simulink model "a01_SimTurret"  (R2024a)
settings: Solver=VariableStepAuto  StartTime=0.0  StopTime=10  FixedStep=0.000001  MaxStep=mSim.dTime*0.01  RelTol=mSim.dTime*0.01
PostLoadFcn:
  | a02_SimVariable
undefined symbols (not defined in the file): A02MTRPA, a1st, B01SCHED, b5th, C01ISENS, c7th, CRX1, DC, E03LIM, H01MDE, H01TRT, Init, mDefine, Mech, mSim, MtrPar, Sim, SIM, SimMde
libraries: spsSeriesRLCBranchLib x17, simulink x8, spsCurrentMeasurementLib x7, spsIGBTDiodeLib x7, spsDiodeLib x6, spsControlledVoltageSourceLib x6, spsVoltageMeasurementLib x4, SignalEditorBlockLib x3, spsDCVoltageSourceLib x1, spspowerguiLib x1
(part 1 of 3)
settings Model: VariantConfigurationObject=cfgVariant  SimulationMode=accelerator  NumberOfSteps=10  Creator=MINV  LastModifiedBy=admin
settings SolverCC: MaxConsecutiveZCs=10000  ZeroCrossAlgorithm=Adaptive  AlgebraicLoopSolver=TrustRegion  AutoInsertRateTranBlk=on
settings DataIOCC: InspectSignalLogs=on
settings OptimizationCC: DefaultParameterBehavior=Inlined  UseDivisionForNetSlopeComputation=UseDivisionForReciprocalsOfIntegersOnly  UseFloatMulNetSlope=on  DefaultUnderspecifiedDataType=single  UseSpecifiedMinMax=on  InlineInvariantSignals=on  EnhancedBackFolding=on  PassReuseOutputArgsAs=Individual arguments  ZeroExternalMemoryAtStartup=off  ZeroInternalMemoryAtStartup=off  NoFixptDivByZeroProtection=on  EfficientFloat2IntCast=on  OptimizeBlockOrder=speed  DifferentSizesBufferReuse=on  OptimizationCustomize=off  EfficientTunableParamExpr=on
settings DebuggingCC: SignalInfNanChecking=warning  MaskedZcDiagnostic=none  IgnoredZcDiagnostic=none  IntegerOverflowMsg=none  ParameterPrecisionLossMsg=none  ParameterTunabilityLossMsg=error  UnconnectedInputMsg=warning  UnconnectedOutputMsg=warning  UnconnectedLineMsg=warning  BusObjectLabelMismatch=error  AssertControl=DisableAll  SFUnexpectedBacktrackingDiag=warning  SFNoUnconditionalDefaultTransitionDiag=warning  SFUndirectedBroadcastEventsDiag=error  SFExecutionAtInitializationDiag=none  UnitsInconsistencyMsg=none  ArithmeticOperatorsInVariantConditions=warning
settings HardwareCC: ProdBitPerPointer=32  ProdBitPerSizeT=32  ProdBitPerPtrDiffT=32  ProdLargestAtomicFloat=None  ProdWordSize=32  ProdHWDeviceType=Infineon->TriCore
settings SFSimCC: SimUseLocalCustomCode=off  CompileTimeRecursionLimit=0  EnableRuntimeRecursion=off  MATLABDynamicMemAlloc=off  CustomCodeUndefinedFunction=UseInterfaceOnly
settings RTWCC: Description=Embedded Coder  SystemTargetFile=ert.tlc  GenCodeOnly=on  TemplateMakefile=ert_default_tmf  GenerateReport=on  RTWUseLocalCustomCode=off  CustomHeaderCode="#include \"Define_ASW_Header.h\""  BuildConfiguration=Faster Runs  IncludeHyperlinkInReport=on  LaunchReport=on  GenerateTraceInfo=on  GPUComputeCapability=3.5  DLArmComputeVersion=19.05
settings RTWCC: CustomTerminator=|
  | mVF.VF_cRef_In = 0.0F;
  |     mVF.VF_cRef_In_z = 0.0F;
  |     mVF.VF_Theta = 0.0F;
  |     mVF.V_cRef_In = 0.0F;
  |     mVF.V_cRef_In_z = 0.0F;
  |     mSr.S_Ref_In = 0.0F;
  |     mSEQ.s_Ref_In_z = 0.0F;
  |     mIr.I_cRef_In = 0.0F;
  |     mIr.I_cRef_In_z = 0.0F;
  |     mIr.I_cRef_Limed_z = 0.0F;
  |     rtDW.I_cRef_Limed = 0.0F;
  | 
  |     // V
  |     mSVP.VRef_Max = 0.0F;
  |     mSVP.VRef_Min = 0.0F;
  |     mVr.Vr_Ref_a = 0.0F;
  |     mVr.Vr_Ref_b = 0.0F;
  |     mVr.Vr_Ref_c = 0.0F;
  |     mVn.Vn_Ref_a = 0.0F;
  |     mVn.Vn_Ref_b = 0.0F;
  |     mVn.Vn_Ref_c = 0.0F;
  |     mVe.Ve_Ref_d = 0.0F;
  |     mVe.Ve_Ref_q = 0.0F;
  |     mVe.Ve_d = 0.0F;
  |     mVe.Ve_q = 0.0F;
  |     mVe.Ve_d_z = 0.0F;
  |     mVe.Ve_q_z = 0.0F;
  | 
  |     // IF Initialize
  |     mMC.IF_FREQ = 0.0F;
  |     mMC.IF_Theta = 0.0F;
  | 
  |     // Current Control Initialize
  |     mVe.Ve_d = 0.0F;
  |     mVe.Ve_q = 0.0F;
  |     mVe.Ve_Ref_d = 0.0F;
  |     mVe.Ve_Ref_q = 0.0F;
  |     mTheta.App_sin = 0.0F;
  |     mTheta.App_cos = 0.0F;
  | 
  |     // Sensorless Sequence
  |     if (mWFlag.Pwm_Action == 0U)
  |     {
  |         mSEQ.STEP = 1U;
  |     }
  | 
  |     // Integ
  |     mInteg.Id_Integ = 0.0F;
  |     mInteg.Iq_Integ = 0.0F;
  |     mInteg.I_cRef_Integ = 0.0F;
  |     mEST.We_Integ = 0.0F;
  |     mEST.We_Integ_z = 0.0F;
  |     mEST.Theta_Integ = 0.0F;
  |     mEST.Theta_z = 0.0F;
  |     mVe.Ve_d = 0.0F;
  |     mSr.S_Ref_In = mSEQ.s_Ref_In_z;
settings CodeAppCC: ForceParamTrailComments=on  IgnoreCustomStorageClasses=off  OperatorAnnotations=on  SimulinkDataObjDesc=on  SFDataObjDesc=on  CustomSymbolStrGlobalVar=rt$N$M  CustomSymbolStrType=$N$M  CustomSymbolStrFcn=$N$M$F  CustomSymbolStrMacro=$N$M  DefineNamingRule=UpperCase  ParamNamingRule=UpperCase  InsertBlockDesc=on  EnableCustomComments=on
settings ERTTargetCC: GenerateSampleERTMain=on  InlinedParameterPlacement=NonHierarchical  ERTCustomFileTemplate=example_file_process.tlc
settings ConfigComp: CovScope=ReferencedModels  CovIncludeTopModel=off  CovMetricSettings=dw  CovSaveCumulativeToWorkspaceVar=on  CovSaveSingleToWorkspaceVar=on  CovExternalEMLEnable=off  PSModelRefIgnoreList=[]  PSEnableModelRefIgnoreList=off  PSModelRefMinMaxVerif=CheckAndConstrain  PSAutoStubLUT=on  DVTestSuiteOptimization=CombinedObjectives (Nonlinear Extended)  DVRebuildModelRepresentation=Always
settings SimscapeCC: SimscapeNormalizeSystem=off

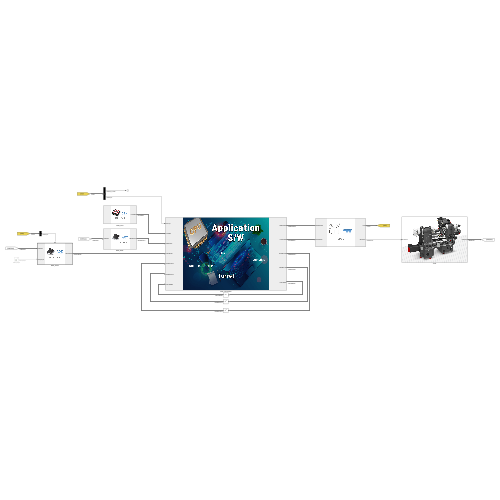
[thumbnail: Simulink's stored preview of the top-level diagram]
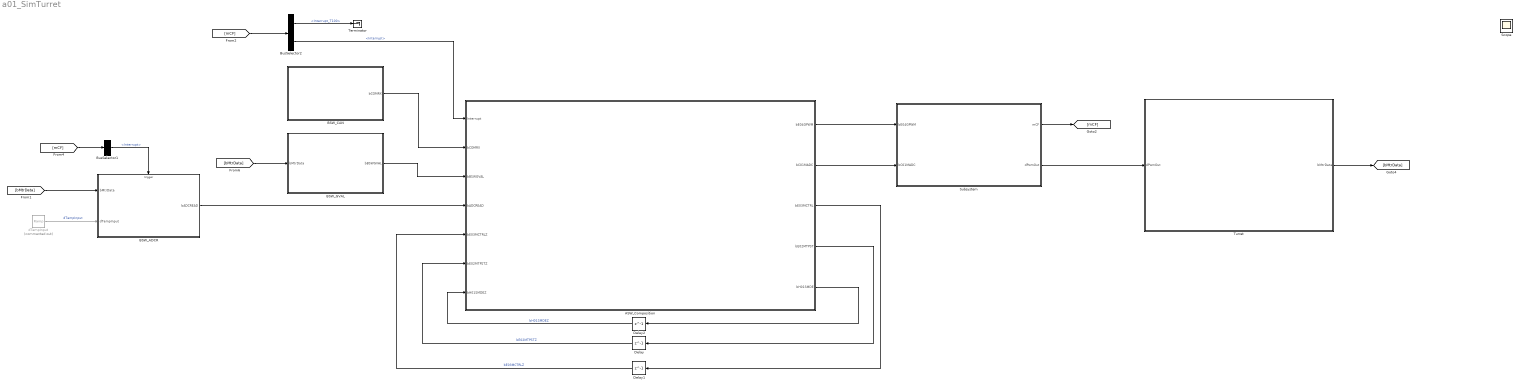
== system a01_SimTurret ==
  ASW_Composition : Subsystem
      mask Display: image('AppSW.png');
  BSW_ADCR : Subsystem
      mask Display: image('ADCREAD_2.png');
  BSW_CAN : Subsystem
      mask Display: image('CANRX1.png');
  BSW_GVAL : Subsystem
      mask Display: image('BSW.png');
  BusSelector1 : BusSelector  OutputSignals=Interrupt
  BusSelector2 : BusSelector  OutputSignals=Interrupt_T100,Interrupt
  Delay : Delay  DelayLength=1
  Delay1 : Delay  DelayLength=1
  Delay2 : Delay  DelayLength=1
  Subsystem : Subsystem
      mask Display: image('ePWM.png');
  Terminator : Terminator
  Turret : Subsystem
      mask Display: image('Turret_2.png');
  dTempInput : simulink/Sources/Ramp  Commented=on  slope=-4096*1.5  start=0  InitialOutput=2048
  Scope : Scope
  wires:
  Turret/1(bMtrData) -> [bMtrData]
  Subsystem/1(mCF) -> [mCF]
  Subsystem/2(dPwmOut) -> Turret/1(dPwmOut)
  [bMtrData] -> BSW_ADCR/1(bMtrData)
  BSW_ADCR/1(bADCREAD) -> ASW_Composition/4(bADCREAD)
  [mCF] -> BusSelector1/1
  BusSelector1/1 -> BSW_ADCR/Trigger  "<Interrupt>"
  dTempInput/1 -> BSW_ADCR/2(dTempInput)  "dTempInput"
  [bMtrData] -> BSW_GVAL/1(bMtrData)
  ASW_Composition/1(bE04GPWM) -> Subsystem/1(bE04GPWM)
  ASW_Composition/2(bC01MADC) -> Subsystem/2(bC01MADC)
  BSW_GVAL/1(bBSWGVAL) -> ASW_Composition/3(bBSWGVAL)
  ASW_Composition/4(bE02MTPST) -> Delay/1
  Delay/1 -> ASW_Composition/6(bE02MTPSTZ)  "bE02MTPSTZ"
  ASW_Composition/3(bE03MCTRL) -> Delay1/1
  Delay1/1 -> ASW_Composition/5(bE03MCTRLZ)  "bE03MCTRLZ"
  BusSelector2/1 -> Terminator/1  "<Interrupt_T100>"
  [mCF] -> BusSelector2/1
  BSW_CAN/1(bCOMRX) -> ASW_Composition/2(bCOMRX)
  ASW_Composition/5(bH01SMDE) -> Delay2/1
  Delay2/1 -> ASW_Composition/7(bH01SMDEZ)  "bH01SMDEZ"
  BusSelector2/2 -> ASW_Composition/1(Interrupt)  "<Interrupt>"

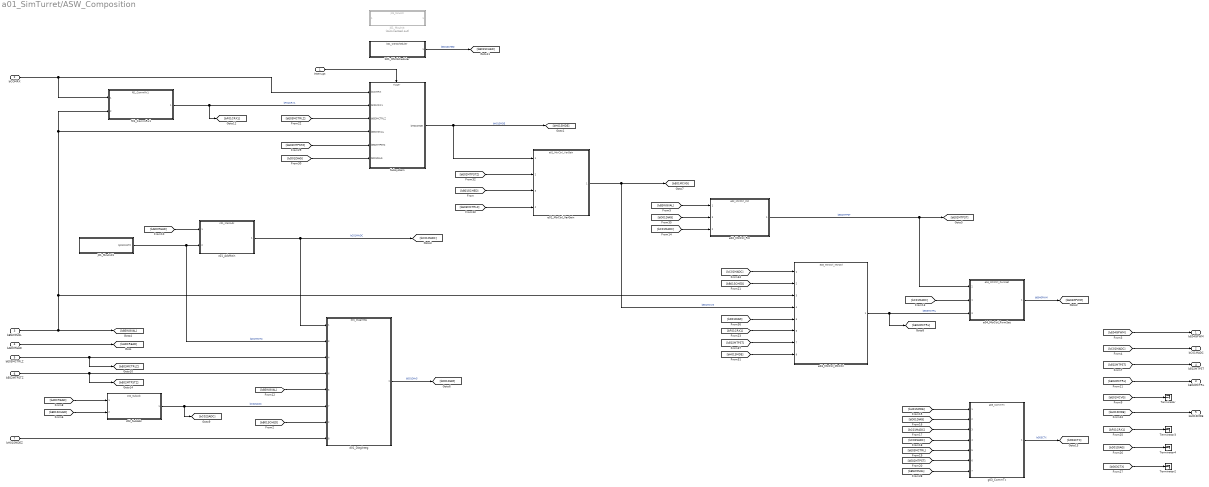
== system a01_SimTurret/ASW_Composition ==
  Interrupt : Inport
  bCOMRX : Inport  Port=2
  bBSWGVAL : Inport  Port=3
  bADCREAD : Inport  Port=4
  bE03MCTRLZ : Inport  Port=5
  bE02MTPSTZ : Inport  Port=6
  bH01SMDEZ : Inport  Port=7
  Subsystem : Subsystem
  Terminator{,2..4} (4 alike) : Terminator
  b01_OSnScheduler : ModelReference  ModelNameDialog=b01_OSnScheduler.slx  SimulationMode=Normal  ModelReferenceVersion=7.234
  c01_AdcMain : ModelReference  ModelNameDialog=c01_MainAdc.slx  SimulationMode=Normal  ModelReferenceVersion=7.199
  c02_SubAdc : ModelReference  ModelNameDialog=c02_SubAdc.slx  SimulationMode=Normal  ModelReferenceVersion=7.333
  d01_Diaglnteg : ModelReference  ModelNameDialog=d01_Diaglnteg.slx  SimulationMode=Normal  ModelReferenceVersion=7.634
      settings: PortSchema="{\"entries\":[{\"content\":{\"sides\":[{\"content\":{\"connectorIds\":[\"In1\",\"In3\",\"In4\",\"In6\",\"In5\",\"In7\",\"In2\",\"In8\"]},\"type\":\"ConnectorPlacement.EquallySpacedRectSide\",\"uuid\":\"173800be-f5dc-4729-8663-94e6b8956988\"},{\"content\":{\"connectorIds\":[\"Out1\"],\"side\":\"RIGHT\"},\"type\":\"ConnectorPlacement.EquallySpacedRectSide\",\"uuid\":\"97fb1ab8-9be5-42b7-b1bf-027aede52d4b\"},{\"content\":{\"side\":\"TOP\"},\"type\":\"ConnectorPlacement.EquallySpacedRectSide\",\"uuid\":\"2e8adbd0-ac2b-453b-9e60-9040db9b7bc5\"}]},\"type\":\"ConnectorPlacement.EquallySpacedConnector\",\"uuid\":\"3d6050df-28eb-4a7c-b004-dbb78ba9bd4d\"}],\"packageUris\":[\"http://schema.mathworks.com/mf0/Connector/R2020b\"],\"version\":\"1.0\"}"
  e01_MtrCtrl_VarGain : ModelReference  ModelNameDialog=e01_MtrCtrl_VarGain.slx  SimulationMode=Normal  ModelReferenceVersion=7.579
  e02_MtrCtrl_Pst : ModelReference  ModelNameDialog=e02_MtrCtrl_Pst.slx  SimulationMode=Normal  ModelReferenceVersion=7.578
      settings: PortSchema="{\"entries\":[{\"content\":{\"sides\":[{\"content\":{\"connectorIds\":[\"In1\",\"In3\",\"In2\"]},\"type\":\"ConnectorPlacement.EquallySpacedRectSide\",\"uuid\":\"f113863a-975d-4050-818f-27abf814cfb5\"},{\"content\":{\"connectorIds\":[\"Out1\"],\"side\":\"RIGHT\"},\"type\":\"ConnectorPlacement.EquallySpacedRectSide\",\"uuid\":\"6686929e-870a-4175-88de-c3673796ef3d\"},{\"content\":{\"side\":\"TOP\"},\"type\":\"ConnectorPlacement.EquallySpacedRectSide\",\"uuid\":\"709e4a9d-e71c-4478-b192-cfc6b94393ff\"}]},\"type\":\"ConnectorPlacement.EquallySpacedConnector\",\"uuid\":\"0b953766-3c3a-41c3-a306-f68929d7ac7c\"}],\"packageUris\":[\"http://schema.mathworks.com/mf0/Connector/R2020b\"],\"version\":\"1.0\"}"
  e03_MtrCtrl_MtrCtrl : ModelReference  ModelNameDialog=e03_MtrCtrl_MtrCtrl.slx  SimulationMode=Normal  ModelReferenceVersion=7.948
  e04_MtrCtrl_PwmSet : ModelReference  ModelNameDialog=e04_MtrCtrl_PwmSet.slx  SimulationMode=Normal  ModelReferenceVersion=7.212
      settings: PortSchema="{\"entries\":[{\"content\":{\"sides\":[{\"content\":{\"connectorIds\":[\"In2\",\"In1\",\"In3\"]},\"type\":\"ConnectorPlacement.EquallySpacedRectSide\",\"uuid\":\"f113863a-975d-4050-818f-27abf814cfb5\"},{\"content\":{\"connectorIds\":[\"Out1\"],\"side\":\"RIGHT\"},\"type\":\"ConnectorPlacement.EquallySpacedRectSide\",\"uuid\":\"6686929e-870a-4175-88de-c3673796ef3d\"},{\"content\":{\"side\":\"TOP\"},\"type\":\"ConnectorPlacement.EquallySpacedRectSide\",\"uuid\":\"709e4a9d-e71c-4478-b192-cfc6b94393ff\"}]},\"type\":\"ConnectorPlacement.EquallySpacedConnector\",\"uuid\":\"0b953766-3c3a-41c3-a306-f68929d7ac7c\"}],\"packageUris\":[\"http://schema.mathworks.com/mf0/Connector/R2020b\"],\"version\":\"1.0\"}"
  f01_CommRx1 : ModelReference  ModelNameDialog=f01_CommRx1.slx  SimulationMode=Normal  ModelReferenceVersion=7.313
  g03_CommTx : ModelReference  ModelNameDialog=g03_CommTx.slx  SimulationMode=Normal  ModelReferenceVersion=7.362
  j01_McuInit : ModelReference  Commented=on  ModelNameDialog=j01_McuInit.slx  SimulationMode=Normal  ModelReferenceVersion=7.616
  j01_McuInit1 : Subsystem
  bE04GPWM : Outport
  bC01MADC : Outport  Port=2
  bE03MCTRL : Outport  Port=3
  bE02MTPST : Outport  Port=4
  bH01SMDE : Outport  Port=5
  wires:
  c01_AdcMain/1 -> [bC01MADC], d01_Diaglnteg/1  "bC01MADC"
  b01_OSnScheduler/1 -> [bB01SCHED]  "bB01SCHED"
  bADCREAD/1 -> [bADCREAD]
  c02_SubAdc/1 -> [bC02SADC], d01_Diaglnteg/7  "bC02SADC"
  e04_MtrCtrl_PwmSet/1 -> [bE04GPWM]  "bE04GPWM"
  [bE04GPWM] -> bE04GPWM/1
  [bC01MADC] -> bC01MADC/1
  e02_MtrCtrl_Pst/1 -> e04_MtrCtrl_PwmSet/2, [bE02MTPST]  "bE02MTPST"
  [bBSWGVAL] -> e02_MtrCtrl_Pst/1
  d01_Diaglnteg/1 -> [bD01DIAG]  "bD01DIAG"
  [bE02MTPST] -> bE02MTPST/1
  e01_MtrCtrl_VarGain/1 -> e03_MtrCtrl_MtrCtrl/4, [bE01MCVG]  "bE01MCVG"
  [bE01MCVG] -> Terminator/1
  bE03MCTRLZ/1 -> [bE03MCTRLZ], d01_Diaglnteg/4
  [bE03MCTRL] -> bE03MCTRL/1
  bE02MTPSTZ/1 -> [bE02MTPSTZ], d01_Diaglnteg/6
  bBSWGVAL/1 -> f01_CommRx1/2, Subsystem/4(bBSWGVAL), e03_MtrCtrl_MtrCtrl/3, [bBSWGVAL]
  [bB01SCHED] -> e01_MtrCtrl_VarGain/3
  [bB01SCHED] -> d01_Diaglnteg/2
  [bB01SCHED] -> c02_SubAdc/2
  [bADCREAD] -> c02_SubAdc/1
  [bADCREAD] -> c01_AdcMain/1
  [bBSWGVAL] -> d01_Diaglnteg/5
  [bC01MADC] -> e04_MtrCtrl_PwmSet/1
  [bC01MADC] -> e02_MtrCtrl_Pst/2
  Subsystem/1(bH01SMDE) -> e01_MtrCtrl_VarGain/1, [bH01SMDE]  "bH01SMDE"
  j01_McuInit1/1(bJ01MINITZ) -> c01_AdcMain/2, d01_Diaglnteg/3  "bJ01MINITZ"
  bCOMRX/1 -> Subsystem/1(bCOMRX), f01_CommRx1/1
  [bF01CRX1] -> e03_MtrCtrl_MtrCtrl/6
  g03_CommTx/1 -> [bG03CTX]  "bG03CTX"
  [bH01SMDE] -> g03_CommTx/1
  [bD01DIAG] -> g03_CommTx/2
  [bC01MADC] -> g03_CommTx/3
  [bE02MTPST] -> g03_CommTx/6
  [bE03MCTRL] -> g03_CommTx/5
  [bC02SADC] -> g03_CommTx/4
  e03_MtrCtrl_MtrCtrl/1 -> e04_MtrCtrl_PwmSet/3, [bE03MCTRL]  "bE03MCTRL"
  [bB01SCHED] -> e03_MtrCtrl_MtrCtrl/2
  [bE03MCTRLZ] -> Subsystem/3(bE03MCTRLZ)
  f01_CommRx1/1 -> [bF01CRX1], Subsystem/2(bF01CRX1)  "bF01CRX1"
  [bH01SMDE] -> bH01SMDE/1
  [bF01CRX1] -> Terminator3/1
  [bD01DIAG] -> Terminator4/1
  [bG03CTX] -> Terminator2/1
  [bBSWGVAL] -> g03_CommTx/7
  [bE02MTPSTZ] -> Subsystem/5(bE02MTPSTZ)
  [bD01DIAG] -> Subsystem/6(bD01DIAG)
  [bH01SMDE] -> e03_MtrCtrl_MtrCtrl/8
  [bE02MTPSTZ] -> e01_MtrCtrl_VarGain/2
  [bE03MCTRLZ] -> e01_MtrCtrl_VarGain/4
  [bC01MADC] -> e03_MtrCtrl_MtrCtrl/1
  [bD01DIAG] -> e02_MtrCtrl_Pst/3
  [bD01DIAG] -> e03_MtrCtrl_MtrCtrl/5
  [bE02MTPST] -> e03_MtrCtrl_MtrCtrl/7
  bH01SMDEZ/1 -> d01_Diaglnteg/8
  Interrupt/1 -> Subsystem/Trigger

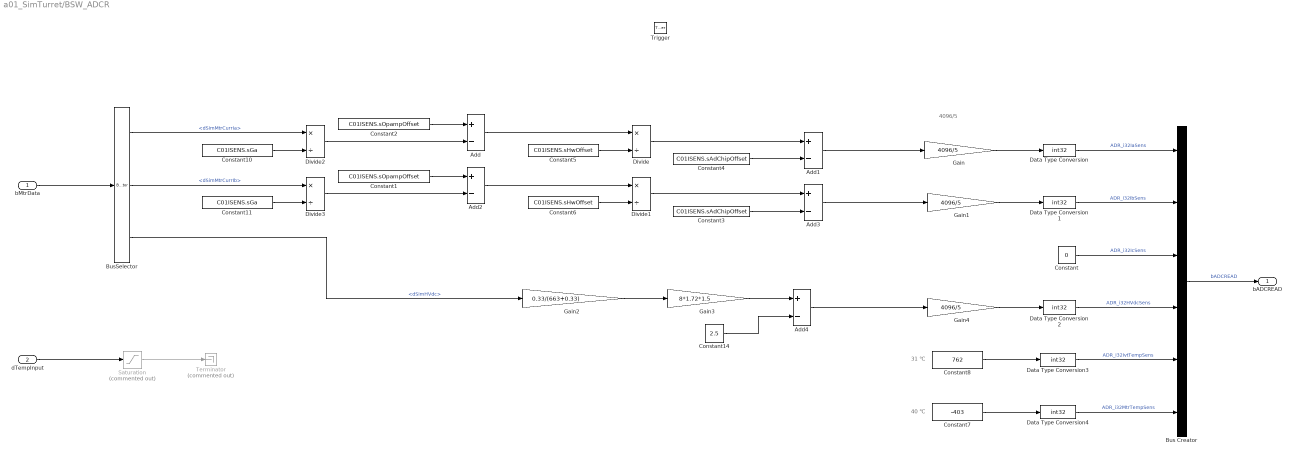
== system a01_SimTurret/BSW_ADCR ==
  note: 4096/5
  note: 40 ℃
  note: 31 ℃
  bMtrData : Inport
  dTempInput : Inport  Port=2
  Trigger : TriggerPort  VariantControl=(inherit)  PortDimensions=1
  Add{,1..4} (5 alike) : Sum  Inputs=+-
  Bus Creator : BusCreator  Inputs=6  OutDataTypeStr=Bus: X_ADCREAD
  BusSelector : BusSelector  OutputSignals=dSimPwrStack.dSimMtrCurrIa,dSimPwrStack.dSimMtrCurrIb,dSimPwrStack.dSimHVdc
  Constant : Constant  Value=0  OutDataTypeStr=int32
  Constant1 : Constant  Value=C01ISENS.sOpampOffset
  Constant10 : Constant  Value=C01ISENS.sGa  OutDataTypeStr=single
  Constant11 : Constant  Value=C01ISENS.sGa  OutDataTypeStr=single
  Constant14 : Constant  Value=2.5
  Constant2 : Constant  Value=C01ISENS.sOpampOffset
  Constant3 : Constant  Value=C01ISENS.sAdChipOffset  OutDataTypeStr=single
  Constant4 : Constant  Value=C01ISENS.sAdChipOffset  OutDataTypeStr=single
  Constant5 : Constant  Value=C01ISENS.sHwOffset  OutDataTypeStr=single
  Constant6 : Constant  Value=C01ISENS.sHwOffset  OutDataTypeStr=single
  Constant7 : Constant  Value=-403
  Constant8 : Constant  Value=762
  Data Type Conversion{,1..4} (5 alike) : DataTypeConversion  OutDataTypeStr=int32  SaturateOnIntegerOverflow=off  RndMeth=Floor
  Divide{,1..3} (4 alike) : Product  Inputs=*/
  Gain : Gain  Gain=4096/5
  Gain1 : Gain  Gain=4096/5
  Gain2 : Gain  Gain=0.33/(663+0.33)
  Gain3 : Gain  Gain=8*1.72*1.5
  Gain4 : Gain  Gain=4096/5
  Saturation : Saturate  Commented=on  UpperLimit=24  LowerLimit=23
  Terminator : Terminator  Commented=on
  bADCREAD : Outport
  wires:
  Constant5/1 -> Divide/2
  Constant2/1 -> Add/1
  Divide/1 -> Add1/1
  Constant4/1 -> Add1/2
  Gain/1 -> Data Type Conversion/1
  Add/1 -> Divide/1
  bMtrData/1 -> BusSelector/1
  BusSelector/1 -> Divide2/1  "<dSimMtrCurrIa>"
  BusSelector/2 -> Divide3/1  "<dSimMtrCurrIb>"
  Bus Creator/1 -> bADCREAD/1  "bADCREAD"
  Data Type Conversion/1 -> Bus Creator/1  "ADR_i32IaSens"
  Constant1/1 -> Add2/1
  Gain1/1 -> Data Type Conversion1/1
  Add2/1 -> Divide1/1
  Constant3/1 -> Add3/2
  Constant6/1 -> Divide1/2
  Divide1/1 -> Add3/1
  Data Type Conversion1/1 -> Bus Creator/2  "ADR_i32IbSens"
  Constant/1 -> Bus Creator/3  "ADR_i32IcSens"
  Gain4/1 -> Data Type Conversion2/1
  Data Type Conversion3/1 -> Bus Creator/5  "ADR_i32IvtTempSens"
  Data Type Conversion4/1 -> Bus Creator/6  "ADR_i32MtrTempSens"
  Constant10/1 -> Divide2/2
  Divide2/1 -> Add/2
  Constant11/1 -> Divide3/2
  Divide3/1 -> Add2/2
  BusSelector/3 -> Gain2/1  "<dSimHVdc>"
  Gain2/1 -> Gain3/1
  Gain3/1 -> Add4/1
  Constant14/1 -> Add4/2
  Add4/1 -> Gain4/1
  Data Type Conversion2/1 -> Bus Creator/4  "ADR_i32HVdcSens"
  dTempInput/1 -> Saturation/1
  Saturation/1 -> Terminator/1
  Constant7/1 -> Data Type Conversion4/1
  Constant8/1 -> Data Type Conversion3/1
  Add1/1 -> Gain/1
  Add3/1 -> Gain1/1

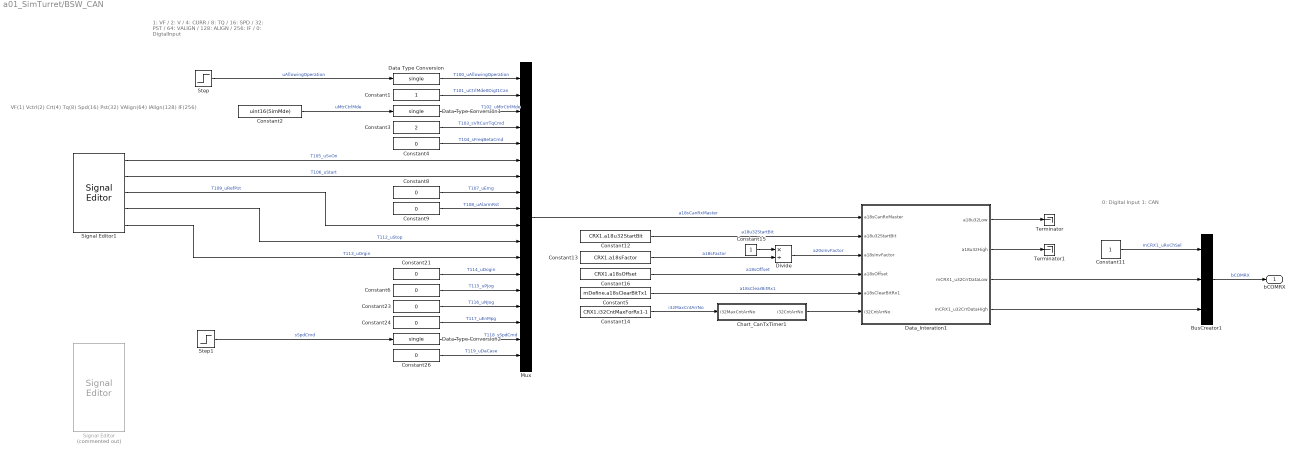
== system a01_SimTurret/BSW_CAN ==
  note: VF(1) Vctrl(2) Crt(4) Tq(8) Spd(16) Pst(32) VAlign(64) IAlign(128) IF(256)
  note: 1: VF / 2: V / 4: CURR / 8: TQ / 16: SPD /
      | 32: PST / 64: VALIGN / 128: ALIGN /
      | 256: IF / 0: DigtalInput
  note: 0: Digital Input
      | 1: CAN
  BusCreator1 : BusCreator  Inputs=3  OutDataTypeStr=Bus: X_COMRX
  Chart_CanTxTimer1 : Stateflow chart  TreatAsAtomicUnit=on
  Constant1 : Constant  OutDataTypeStr=single
  Constant11 : Constant  OutDataTypeStr=uint16
  Constant12 : Constant  Value=CRX1.a18u32StartBit
  Constant13 : Constant  Value=CRX1.a18sFactor
  Constant14 : Constant  Value=CRX1.i32CntMaxForRx1-1  OutDataTypeStr=int32
  Constant15 : Constant  OutDataTypeStr=single
  Constant16 : Constant  Value=CRX1.a18sOffset
  Constant2 : Constant  Value=uint16(SimMde)  OutDataTypeStr=single
  Constant{4,6,8..9,21,23..24,26} (8 alike) : Constant  Value=0  OutDataTypeStr=single
  Constant3 : Constant  Value=2  OutDataTypeStr=single
  Constant5 : Constant  Value=mDefine.a18sClearBitTx1
  Data Type Conversion : DataTypeConversion  OutDataTypeStr=single  SaturateOnIntegerOverflow=off  RndMeth=Floor
  Data Type Conversion1 : DataTypeConversion  OutDataTypeStr=single  SaturateOnIntegerOverflow=off  RndMeth=Floor
  Data Type Conversion2 : DataTypeConversion  OutDataTypeStr=single  SaturateOnIntegerOverflow=off  RndMeth=Floor
  Data_Interation1 : Stateflow chart  TreatAsAtomicUnit=on
      settings: RTWSystemCode=Inline
  Divide : Product  Inputs=*/  OutDataTypeStr=single
  Mux : Mux  Inputs=18
  Signal Editor : SignalEditorBlockLib/Signal Editor  Commented=on  FileName=TestOrigin3.mat  ActiveScenario=Scenario  ActiveSignal=Origin  IsBus=off  OutputBusObjectStr=Bus: BusObject  SampleTime=0  Interpolate=off  ZeroCross=off  OutputAfterFinalValue=Setting to zero  Unit=inherit  PreserveSignalName=on  ApplySigPropsToAllScenarios=on  ApplySigPropsToAllSignals=off
  Signal Editor1 : SignalEditorBlockLib/Signal Editor  FileName=TestOrigin4.mat  ActiveScenario=Scenario  ActiveSignal=Origin  IsBus=off  OutputBusObjectStr=Bus: BusObject  SampleTime=0  Interpolate=off  ZeroCross=off  OutputAfterFinalValue=Setting to zero  Unit=inherit  PreserveSignalName=on  ApplySigPropsToAllScenarios=on  ApplySigPropsToAllSignals=off
  Step : Step  After=0  SampleTime=0
  Step1 : Step  Time=3  Before=-500  After=1000  SampleTime=0
  Terminator : Terminator
  Terminator1 : Terminator
  bCOMRX : Outport
  wires:
  Constant5/1 -> Data_Interation1/5(a18sClearBitRx1)  "a18sClearBitRx1"
  Data_Interation1/4(mCRX1_u32CrrDataHigh) -> BusCreator1/3
  Constant13/1 -> Divide/2  "a18sFactor"
  Mux/1 -> Data_Interation1/1(a18sCanRxMaster)  "a18sCanRxMaster"
  Constant14/1 -> Chart_CanTxTimer1/1(i32MaxCntArrNo)  "i32MaxCntArrNo"
  Divide/1 -> Data_Interation1/3(a18sInvFactor)  "a20sInvFactor"
  Data_Interation1/1(a18u32Low) -> Terminator/1
  Data_Interation1/2(a18u32High) -> Terminator1/1
  Constant12/1 -> Data_Interation1/2(a18u32StartBit)  "a18u32StartBit"
  Data_Interation1/3(mCRX1_u32CrrDataLow) -> BusCreator1/2
  Constant16/1 -> Data_Interation1/4(a18sOffset)  "a18sOffset"
  Chart_CanTxTimer1/1(i32CntArrNo) -> Data_Interation1/6(i32CntArrNo)
  BusCreator1/1 -> bCOMRX/1  "bCOMRX"
  Constant15/1 -> Divide/1
  Constant11/1 -> BusCreator1/1  "mCRX1_uRxChSel"
  Data Type Conversion/1 -> Mux/1  "T100_uAllowingOperation"
  Constant1/1 -> Mux/2  "T101_uCtrlMde0Digt1Can"
  Constant2/1 -> Data Type Conversion1/1  "uMtrCtrlMde"
  Constant3/1 -> Mux/4  "T103_sVltCurrTqCmd"
  Constant8/1 -> Mux/8  "T107_uEmg"
  Signal Editor1/2 -> Mux/7  "T106_uStart"
  Signal Editor1/1 -> Mux/6  "T105_uSvOn"
  Constant4/1 -> Mux/5  "T104_sFreqBetaCmd"
  Signal Editor1/4 -> Mux/11  "T112_uStop"
  Signal Editor1/5 -> Mux/12  "T113_uOrgin"
  Constant21/1 -> Mux/13  "T114_uDogin"
  Constant6/1 -> Mux/14  "T115_uPJog"
  Signal Editor1/3 -> Mux/10  "T109_uRefPst"
  Constant9/1 -> Mux/9  "T108_uAlarmRst"
  Constant23/1 -> Mux/15  "T116_uNJog"
  Constant26/1 -> Mux/18  "T119_uDaCase"
  Constant24/1 -> Mux/16  "T117_uEnMpg"
  Data Type Conversion1/1 -> Mux/3  "T102_uMtrCtrlMde"
  Data Type Conversion2/1 -> Mux/17  "T118_sSpdCmd"
  Step/1 -> Data Type Conversion/1  "uAllowingOperation"
  Step1/1 -> Data Type Conversion2/1  "sSpdCmd"

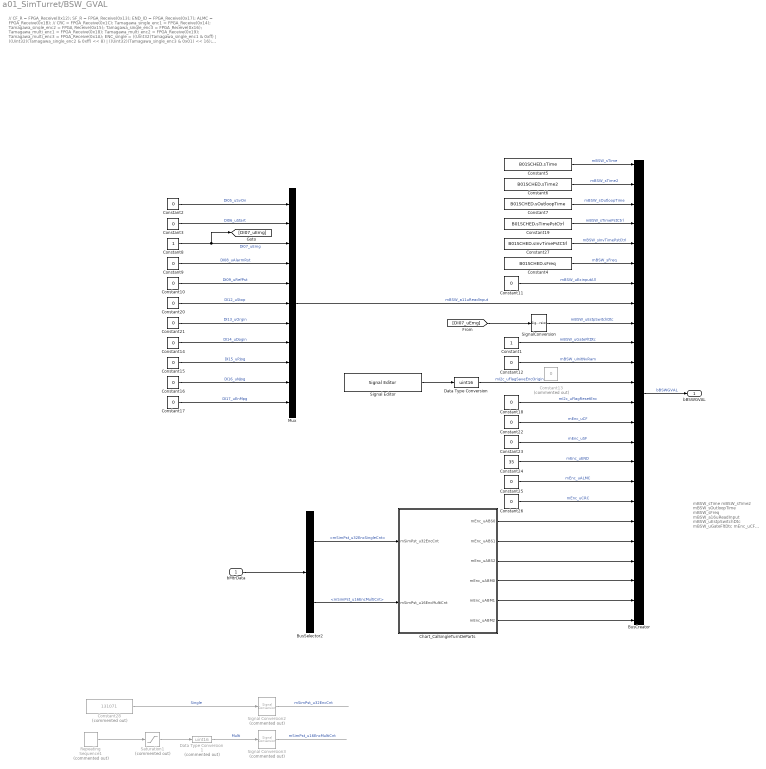
== system a01_SimTurret/BSW_GVAL ==
  note: mBSW_sTime
      |  mBSW_sTime2
      |  mBSW_sOutloopTime
      |  mBSW_sFreq
      |  mBSW_a16uReadInput
      |  mBSW_uEstpSwitchDtc
      |  mBSW_uGateFltDtc
      |  mEnc_uCF
      |  mEnc_uSF
      |  mEnc_uEND
      |  mEnc_uALMC
      |  mEnc_uCRC
      |  mEnc_uABS0
      |  mEnc_uABS1
      |  mEnc_uABS2
      |  mEnc_uABM0
      |  mEnc_uABM1
      |  mEnc_uABM2
  note: // CF_R = FPGA_Receive(0x12);
      |    SF_R = FPGA_Receive(0x13);
      |    END_ID = FPGA_Receive(0x17);
      |    ALMC = FPGA_Receive(0x1B);
      | // CRC = FPGA_Receive(0x1C);
      |
      | Tamagawa_single_enc1 = FPGA_Receive(0x14);
      | Tamagawa_single_enc2 = FPGA_Receive(0x15);
      | Tamagawa_single_enc3 = FPGA_Receive(0x16);
      | Tamagawa_multi_enc1 = FPGA_Receive(0x18);
      | Tamagawa_multi_enc2 = FPGA_Receive(0x19);
      | Tamagawa_multi_enc3 = FPGA_Receive(0x1A);
      |
      | ENC_single = ((Uint32)Tamagawa_single_enc1 & 0xff) | ((Uint32)(Tamagawa_single_enc2 & 0xff) << 8) | ((Uint32)(Tamagawa_single_enc3 & 0x01) << 16);
      | ENC_multi_ORI = ((Uint32)Tamagawa_multi_enc1 & 0xff) | ((Uint32)(Tamagawa_multi_enc2 & 0xff) << 8) | ((Uint32)(Tamagawa_multi_enc3 & 0x01) << 16);
      |
      | if(ENC_multi_ORI > MULTI_OFFSET)
      | 	ENC_multi = ENC_multi_ORI - MULTI_OFFSET;
      | else
      | 	ENC_multi = ENC_multi_ORI + MULTI_OFFSET;
      |
      | Position = ((Uint64)ENC_single & 0x0001ffff) | ((Uint64)(ENC_multi & 0x0000ffff) << 17);
  bMtrData : Inport
  BusCreator : BusCreator  Inputs=24  OutDataTypeStr=Bus: X_BSWGVAL
  BusSelector2 : BusSelector  OutputSignals=bSimMtr.mSimPst_u32EncSingleCnt,bSimMtr.mSimPst_u16EncMultiCnt
  Chart_CalSingleTurnDeParts : Stateflow chart  TreatAsAtomicUnit=on
  Constant1 : Constant  OutDataTypeStr=uint16
  Constant{2..3,9..12,14..18,20..23,25..26} (17 alike) : Constant  Value=0  OutDataTypeStr=uint16
  Constant13 : Constant  Commented=on  Value=0  OutDataTypeStr=uint16
  Constant19 : Constant  Value=B01SCHED.sTimePstCtrl
  Constant24 : Constant  Value=35  OutDataTypeStr=uint16
  Constant27 : Constant  Value=B01SCHED.sInvTimePstCtrl
  Constant28 : Constant  Commented=on  Value=131071  OutDataTypeStr=uint32
  Constant4 : Constant  Value=B01SCHED.sFreq
  Constant5 : Constant  Value=B01SCHED.sTime
  Constant6 : Constant  Value=B01SCHED.sTime2
  Constant7 : Constant  Value=B01SCHED.sOutloopTime
  Constant8 : Constant  OutDataTypeStr=uint16
  Data Type Conversion : DataTypeConversion  OutDataTypeStr=uint16  SaturateOnIntegerOverflow=off  RndMeth=Floor
  Data Type Conversion1 : DataTypeConversion  Commented=on  OutDataTypeStr=uint16  SaturateOnIntegerOverflow=off  RndMeth=Floor
  Mux : Mux  Inputs=11
  Repeating Sequence1 : simulink/Sources/Repeating Sequence  Commented=on  rep_seq_t=[0 0.5]  rep_seq_y=[0 65535]
  Saturation1 : Saturate  Commented=on  UpperLimit=65535  LowerLimit=0
  Signal Conversion2 : SignalConversion  Commented=on  OverrideOpt=off
  Signal Conversion3 : SignalConversion  Commented=on  OverrideOpt=off
  Signal Editor : SignalEditorBlockLib/Signal Editor  FileName=TestOrigin_I2C.mat  ActiveScenario=Scenario1  ActiveSignal=mI2c_uFlagSaveEncOrigin  IsBus=off  OutputBusObjectStr=Bus: BusObject  SampleTime=0  Interpolate=off  ZeroCross=off  OutputAfterFinalValue=Setting to zero  Unit=inherit  PreserveSignalName=on  ApplySigPropsToAllScenarios=on  ApplySigPropsToAllSignals=off
  SignalConversion : SignalConversion  OverrideOpt=off
  bBSWGVAL : Outport
  wires:
  Constant7/1 -> BusCreator/3  "mBSW_sOutloopTime"
  Constant6/1 -> BusCreator/2  "mBSW_sTime2"
  Constant4/1 -> BusCreator/6  "mBSW_sFreq"
  Constant5/1 -> BusCreator/1  "mBSW_sTime"
  BusCreator/1 -> bBSWGVAL/1  "bBSWGVAL"
  bMtrData/1 -> BusSelector2/1
  SignalConversion/1 -> BusCreator/9  "mBSW_uEstpSwitchDtc"
  Constant1/1 -> BusCreator/10  "mBSW_uGateFltDtc"
  Mux/1 -> BusCreator/8  "mBSW_a11uReadInput"
  Constant2/1 -> Mux/1  "DI05_uSvOn"
  Constant3/1 -> Mux/2  "DI06_uStart"
  Constant8/1 -> [DI07_uEmg], Mux/3  "DI07_uEmg"
  Constant9/1 -> Mux/4  "DI08_uAlarmRst"
  Constant10/1 -> Mux/5  "DI09_uRefPst"
  Constant20/1 -> Mux/6  "DI12_uStop"
  Constant21/1 -> Mux/7  "DI13_uOrgin"
  Constant14/1 -> Mux/8  "DI14_uDogin"
  Constant15/1 -> Mux/9  "DI15_uPJog"
  Constant16/1 -> Mux/10  "DI16_uNJog"
  Constant17/1 -> Mux/11  "DI17_uEnMpg"
  Constant22/1 -> BusCreator/14  "mEnc_uCF"
  Constant23/1 -> BusCreator/15  "mEnc_uSF"
  Constant25/1 -> BusCreator/17  "mEnc_uALMC"
  Constant24/1 -> BusCreator/16  "mEnc_uEND"
  Chart_CalSingleTurnDeParts/2(mEnc_uABS1) -> BusCreator/20
  Chart_CalSingleTurnDeParts/3(mEnc_uABS2) -> BusCreator/21
  Chart_CalSingleTurnDeParts/1(mEnc_uABS0) -> BusCreator/19
  Constant26/1 -> BusCreator/18  "mEnc_uCRC"
  BusSelector2/2 -> Chart_CalSingleTurnDeParts/2(mSimPst_u16EncMultiCnt)  "<mSimPst_u16EncMultiCnt>"
  Chart_CalSingleTurnDeParts/4(mEnc_uABM0) -> BusCreator/22
  Chart_CalSingleTurnDeParts/5(mEnc_uABM1) -> BusCreator/23
  Chart_CalSingleTurnDeParts/6(mEnc_uABM2) -> BusCreator/24
  Signal Conversion3/1 -> ?  "mSimPst_u16EncMultiCnt"
  Signal Conversion2/1 -> ?  "mSimPst_u32EncCnt"
  Data Type Conversion1/1 -> Signal Conversion3/1  "Multi"
  Saturation1/1 -> Data Type Conversion1/1
  Repeating Sequence1/1 -> Saturation1/1
  Constant28/1 -> Signal Conversion2/1  "Single"
  BusSelector2/1 -> Chart_CalSingleTurnDeParts/1(mSimPst_u32EncCnt)  "<mSimPst_u32EncSingleCnt>"
  [DI07_uEmg] -> SignalConversion/1
  Constant11/1 -> BusCreator/7  "mBSW_uExinputAll"
  Constant12/1 -> BusCreator/11  "mBSW_uInitNvRam"
  Data Type Conversion/1 -> BusCreator/12  "mI2c_uFlagSaveEncOrigin"
  Constant18/1 -> BusCreator/13  "mI2c_uFlagResetEnc"
  Signal Editor/1 -> Data Type Conversion/1
  Constant19/1 -> BusCreator/4  "mBSW_sTimePstCtrl"
  Constant27/1 -> BusCreator/5  "mBSW_sInvTimePstCtrl"

== system a01_SimTurret/Subsystem ==
  bE04GPWM : Inport
  bC01MADC : Inport  Port=2
  Bus Selector : BusSelector  OutputSignals=Interrupt
  Ftn_BswLayer : Subsystem
  Ftn_MtrCtrlPwmSet : Subsystem
  Interrupt_BSW : Subsystem
      mask Display: image('$imagefile'); % 변경하려면 툴스트립에 있는 "이미지 편집"을 사용하십시오.
  mCF : Outport
  dPwmOut : Outport  Port=2
  wires:
  Ftn_BswLayer/1(dPwmOut) -> dPwmOut/1
  Bus Selector/1 -> Ftn_MtrCtrlPwmSet/Trigger  "<Interrupt>"
  bE04GPWM/1 -> Ftn_MtrCtrlPwmSet/2(bE04GPWM)
  bC01MADC/1 -> Ftn_MtrCtrlPwmSet/1(bC01MADC)
  Ftn_MtrCtrlPwmSet/1(uPwmCompVal) -> Ftn_BswLayer/2(uPwmCompVal)
  Ftn_MtrCtrlPwmSet/2(uPwmOut) -> Ftn_BswLayer/3(uPwmOut)
  Interrupt_BSW/1(mCF) -> mCF/1, Ftn_BswLayer/1(mCF), Bus Selector/1

== system a01_SimTurret/Turret ==
  dPwmOut : Inport
  Inverter : Subsystem
      mask Display: image('SERVO.png');
  SimFtnServoMotor : Subsystem
      mask Display: image('Image04_ServoMotor.png'); % 변경하려면 툴스트립에 있는 "이미지 편집"을 사용하십시오.
  SystemLoad : Subsystem
      mask Display: image('Turret_1.jpg');
  bMtrData : Outport
  wires:
  dPwmOut/1 -> Inverter/1(dPwmOut)
  SimFtnServoMotor/1(bMtrData) -> [bMtrData], bMtrData/1
  SystemLoad/2(S_Load) -> SimFtnServoMotor/2(S_Load)
  SystemLoad/1(T_Load) -> SimFtnServoMotor/1(T_Load)
  Inverter/1(dSimPwrStack) -> SimFtnServoMotor/3(dSimPwrStack)
  [bMtrData] -> SystemLoad/1(bMtrData)
  connections:
  SimFtnServoMotor/LConn3 -- Inverter/RConn3
  SimFtnServoMotor/LConn2 -- Inverter/RConn2
  SimFtnServoMotor/LConn1 -- Inverter/RConn1

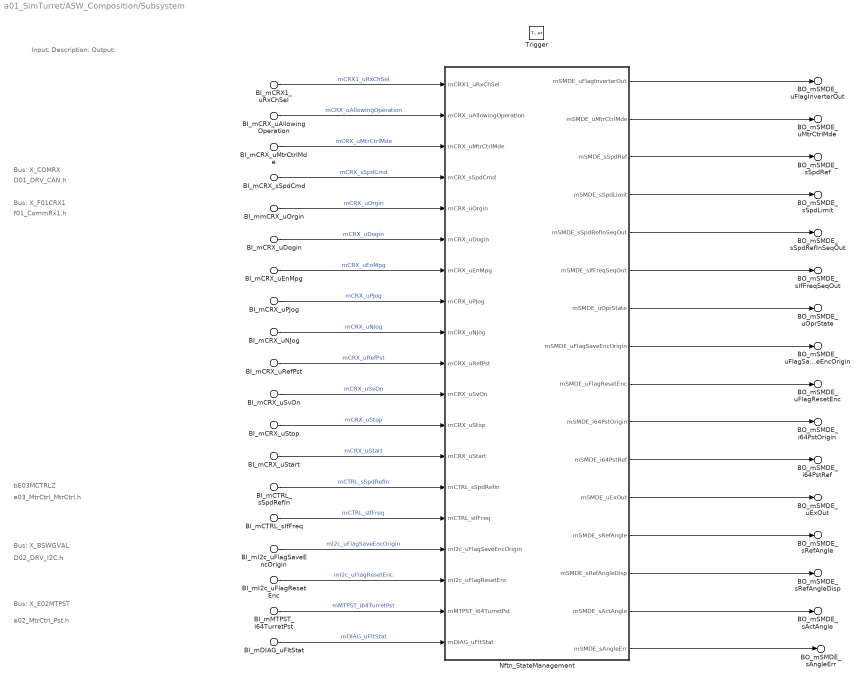
== system a01_SimTurret/ASW_Composition/Subsystem ==
  note: bE03MCTRLZ
  note: e02_MtrCtrl_Pst.h
  note: e03_MtrCtrl_MtrCtrl.h
  note: f01_CommRx1.h
  note: D01_DRV_CAN.h
  note: D02_DRV_I2C.h
  note: Bus: X_BSWGVAL
  note: Bus: X_COMRX
  note: Bus: X_F01CRX1
  note: Input:
      | Description:
      | Output:
  note: Bus: X_E02MTPST
  BI_mCRX1_uRxChSel : Inport  PortName=bCOMRX  Element=mCRX1_uRxChSel
  BI_mCRX_uAllowingOperation : Inport  Port=2  PortName=bF01CRX1  Element=mCRX_uAllowingOperation
  BI_mCRX_uMtrCtrlMde : Inport  Port=2  PortName=bF01CRX1  Element=mCRX_uMtrCtrlMde
  BI_mCRX_uStart : Inport  Port=2  PortName=bF01CRX1  Element=mCRX_uStart
  BI_mCRX_uRefPst : Inport  Port=2  PortName=bF01CRX1  Element=mCRX_uRefPst
  BI_mmCRX_uOrgin : Inport  Port=2  PortName=bF01CRX1  Element=mCRX_uOrgin
  BI_mCRX_uDogin : Inport  Port=2  PortName=bF01CRX1  Element=mCRX_uDogin
  BI_mCRX_uPJog : Inport  Port=2  PortName=bF01CRX1  Element=mCRX_uPJog
  BI_mCRX_uNJog : Inport  Port=2  PortName=bF01CRX1  Element=mCRX_uNJog
  BI_mCRX_uEnMpg : Inport  Port=2  PortName=bF01CRX1  Element=mCRX_uEnMpg
  BI_mCRX_sSpdCmd : Inport  Port=2  PortName=bF01CRX1  Element=mCRX_sSpdCmd
  BI_mCRX_uSvOn : Inport  Port=2  PortName=bF01CRX1  Element=mCRX_uSvOn
  BI_mCRX_uStop : Inport  Port=2  PortName=bF01CRX1  Element=mCRX_uStop
  BI_mCTRL_sIfFreq : Inport  Description=■ 설명: IF Control Frequency  Port=3  PortName=bE03MCTRLZ  Element=mCTRL_sIfFreq
  BI_mCTRL_sSpdRefIn : Inport  Description=■ 설명: 속도 Slop 지령  Port=3  PortName=bE03MCTRLZ  Element=mCTRL_sSpdRefIn
  BI_mI2c_uFlagSaveEncOrigin : Inport  Description=■ 설명: 엔코더 원점 저장 활성화 신호  Port=4  PortName=bBSWGVAL  Element=mI2c_uFlagSaveEncOrigin
  BI_mI2c_uFlagResetEnc : Inport  Description=■ 설명: 엔코더 멀티턴 리셋 활성화 신호  Port=4  PortName=bBSWGVAL  Element=mI2c_uFlagResetEnc
  BI_mMTPST_i64TurretPst : Inport  Description=■ 설명: Turret Position  Port=5  PortName=bE02MTPSTZ  Element=mMTPST_i64TurretPst
  BI_mDIAG_uFltStat : Inport  Description=■ 설명: 고장 신호 대표 값  Port=6  PortName=bD01DIAG  Element=mDIAG_uFltStat
  Trigger : TriggerPort  VariantControl=(inherit)  PortDimensions=1
  Nftn_StateManagement : Subsystem
  BO_mSMDE_uFlagInverterOut : Outport  Description=■ 설명: Allow Operation 신호 (0: 구정 정지, 1: 구동)  PortName=bH01SMDE  Element=mSMDE_uFlagInverterOut
  BO_mSMDE_sSpdRefInSeqOut : Outport  Description=■ 설명: Speed Slop 제어를 위한 이전 지령 속도  PortName=bH01SMDE  Element=mSMDE_sSpdRefInSeqOut
  BO_mSMDE_sSpdLimit : Outport  Description=■ 설명: 속도 제한값  PortName=bH01SMDE  Element=mSMDE_sSpdLimit
  BO_mSMDE_sSpdRef : Outport  Description=■ 설명: 속도 지령  PortName=bH01SMDE  Element=mSMDE_sSpdRef
  BO_mSMDE_sIfFreqSeqOut : Outport  Description=■ 설명: 모터 구동 모드 (0_IO/1_VF/2_V/4_CURR/8_TQ/16_SPD/32_PST/64_VALIGN/128_ALIGN/256_IF)  PortName=bH01SMDE  Element=mSMDE_sIfFreqSeqOut
  BO_mSMDE_uMtrCtrlMde : Outport  Description=■ 설명: 운영 모드 (모터 구동 모드)  PortName=bH01SMDE  Element=mSMDE_uMtrCtrlMde
  BO_mSMDE_uOprState : Outport  Description=■ 설명: 운영 모드 (1H : Standby / 2H : JOG / 4H : MPG_JOG / 8H: Operating / 16H : Wait / 32H: Origin)  PortName=bH01SMDE  Element=mSMDE_uOprState
  BO_mSMDE_uFlagSaveEncOrigin : Outport  Description=■ 설명: 엔코더 원점 저장 활성화 신호  PortName=bH01SMDE  Element=mSMDE_uFlagSaveEncOrigin
  BO_mSMDE_uFlagResetEnc : Outport  Description=■ 설명: 엔코더 멀티턴 리셋 활성화 신호  PortName=bH01SMDE  Element=mSMDE_uFlagResetEnc
  BO_mSMDE_i64PstOrigin : Outport  Description=■ 설명: Encoder 원점 정보  PortName=bH01SMDE  Element=mSMDE_i64PstOrigin
  BO_mSMDE_i64PstRef : Outport  Description=■ 설명: Position Reference  PortName=bH01SMDE  Element=mSMDE_i64PstRef
  BO_mSMDE_sRefAngle : Outport  Description=■ 설명: 터렛 지령 위치  PortName=bH01SMDE  Element=mSMDE_sRefAngle
  BO_mSMDE_sRefAngleDisp : Outport  Description=■ 설명: 터렛 지령 위치 모니터 값 (0~ 360deg로 변환)  PortName=bH01SMDE  Element=mSMDE_sRefAngleDisp
  BO_mSMDE_sActAngle : Outport  Description=■ 설명: 터렛 현재 위치  PortName=bH01SMDE  Element=mSMDE_sActAngle
  BO_mSMDE_sAngleErr : Outport  Description=■ 설명: 터렛 위치 오차  PortName=bH01SMDE  Element=mSMDE_sAngleErr
  BO_mSMDE_uExOut : Outport  PortName=bH01SMDE  Element=mSMDE_uExOut
  wires:
  Nftn_StateManagement/3(mSMDE_sSpdRef) -> BO_mSMDE_sSpdRef/1
  Nftn_StateManagement/11(mSMDE_i64PstRef) -> BO_mSMDE_i64PstRef/1
  Nftn_StateManagement/12(mSMDE_uExOut) -> BO_mSMDE_uExOut/1
  BI_mCRX_uRefPst/1 -> Nftn_StateManagement/10(mCRX_uRefPst)  "mCRX_uRefPst"
  BI_mCRX_uEnMpg/1 -> Nftn_StateManagement/7(mCRX_uEnMpg)  "mCRX_uEnMpg"
  BI_mCRX_uNJog/1 -> Nftn_StateManagement/9(mCRX_uNJog)  "mCRX_uNJog"
  BI_mCRX_uPJog/1 -> Nftn_StateManagement/8(mCRX_uPJog)  "mCRX_uPJog"
  BI_mDIAG_uFltStat/1 -> Nftn_StateManagement/19(mDIAG_uFltStat)  "mDIAG_uFltStat"
  Nftn_StateManagement/10(mSMDE_i64PstOrigin) -> BO_mSMDE_i64PstOrigin/1
  BI_mI2c_uFlagResetEnc/1 -> Nftn_StateManagement/17(mI2c_uFlagResetEnc)  "mI2c_uFlagResetEnc"
  BI_mCRX_uStart/1 -> Nftn_StateManagement/13(mCRX_uStart)  "mCRX_uStart"
  BI_mCTRL_sSpdRefIn/1 -> Nftn_StateManagement/14(mCTRL_sSpdRefIn)  "mCTRL_sSpdRefIn"
  BI_mI2c_uFlagSaveEncOrigin/1 -> Nftn_StateManagement/16(mI2c_uFlagSaveEncOrigin)  "mI2c_uFlagSaveEncOrigin"
  Nftn_StateManagement/9(mSMDE_uFlagResetEnc) -> BO_mSMDE_uFlagResetEnc/1
  BI_mMTPST_i64TurretPst/1 -> Nftn_StateManagement/18(mMTPST_i64TurretPst)  "mMTPST_i64TurretPst"
  BI_mCRX_uAllowingOperation/1 -> Nftn_StateManagement/2(mCRX_uAllowingOperation)  "mCRX_uAllowingOperation"
  Nftn_StateManagement/5(mSMDE_sSpdRefInSeqOut) -> BO_mSMDE_sSpdRefInSeqOut/1
  BI_mCRX_uDogin/1 -> Nftn_StateManagement/6(mCRX_uDogin)  "mCRX_uDogin"
  Nftn_StateManagement/8(mSMDE_uFlagSaveEncOrigin) -> BO_mSMDE_uFlagSaveEncOrigin/1
  Nftn_StateManagement/2(mSMDE_uMtrCtrlMde) -> BO_mSMDE_uMtrCtrlMde/1
  BI_mmCRX_uOrgin/1 -> Nftn_StateManagement/5(mCRX_uOrgin)  "mCRX_uOrgin"
  BI_mCRX1_uRxChSel/1 -> Nftn_StateManagement/1(mCRX1_uRxChSel)  "mCRX1_uRxChSel"
  BI_mCTRL_sIfFreq/1 -> Nftn_StateManagement/15(mCTRL_sIfFreq)  "mCTRL_sIfFreq"
  Nftn_StateManagement/7(mSMDE_uOprState) -> BO_mSMDE_uOprState/1
  Nftn_StateManagement/6(mSMDE_sIfFreqSeqOut) -> BO_mSMDE_sIfFreqSeqOut/1
  Nftn_StateManagement/1(mSMDE_uFlagInverterOut) -> BO_mSMDE_uFlagInverterOut/1
  BI_mCRX_sSpdCmd/1 -> Nftn_StateManagement/4(mCRX_sSpdCmd)  "mCRX_sSpdCmd"
  BI_mCRX_uMtrCtrlMde/1 -> Nftn_StateManagement/3(mCRX_uMtrCtrlMde)  "mCRX_uMtrCtrlMde"
  BI_mCRX_uSvOn/1 -> Nftn_StateManagement/11(mCRX_uSvOn)  "mCRX_uSvOn"
  Nftn_StateManagement/13(mSMDE_sRefAngle) -> BO_mSMDE_sRefAngle/1
  Nftn_StateManagement/15(mSMDE_sActAngle) -> BO_mSMDE_sActAngle/1
  Nftn_StateManagement/16(mSMDE_sAngleErr) -> BO_mSMDE_sAngleErr/1
  BI_mCRX_uStop/1 -> Nftn_StateManagement/12(mCRX_uStop)  "mCRX_uStop"
  Nftn_StateManagement/4(mSMDE_sSpdLimit) -> BO_mSMDE_sSpdLimit/1
  Nftn_StateManagement/14(mSMDE_sRefAngleDisp) -> BO_mSMDE_sRefAngleDisp/1

== system a01_SimTurret/ASW_Composition/j01_McuInit1 ==
  note: Input:
      | ▷
      | Description:
      | ▷
      | Output:
      | ▷
  Constant : Constant  Value=0  OutDataTypeStr=single
  Constant1 : Constant  Value=0  OutDataTypeStr=single
  Constant2 : Constant  Value=0  OutDataTypeStr=uint16
  Constant3 : Constant  Value=0  OutDataTypeStr=uint16
  BO_mMinit_sCurrOfsIa : Outport  Description=■ 설명: A상 전류 센서 오프셋  PortName=bJ01MINITZ  Element=mMinit_sCurrOfsIa
  BO_mMinit_sCurrOfsIb : Outport  Description=■ 설명: B상 전류 센서 오프셋  PortName=bJ01MINITZ  Element=mMinit_sCurrOfsIb
  BO_mMinit_uFlgChangeISR : Outport  Description=■ 설명: 인터럽트 변경 Flag  PortName=bJ01MINITZ  Element=mMinit_uFlgChangeISR
  BO_mMinit_uHwFltCurrOffset : Outport  Description=■ 설명: 전류 센서 오프셋 고장 신호  PortName=bJ01MINITZ  Element=mMinit_uHwFltCurrOffset
  wires:
  Constant/1 -> BO_mMinit_sCurrOfsIa/1  "mMinit_sCurrOfsIa"
  Constant1/1 -> BO_mMinit_sCurrOfsIb/1  "mMinit_sCurrOfsIb"
  Constant2/1 -> BO_mMinit_uFlgChangeISR/1  "mMinit_uFlgChangeISR"
  Constant3/1 -> BO_mMinit_uHwFltCurrOffset/1  "mMinit_uHwFltCurrOffset"

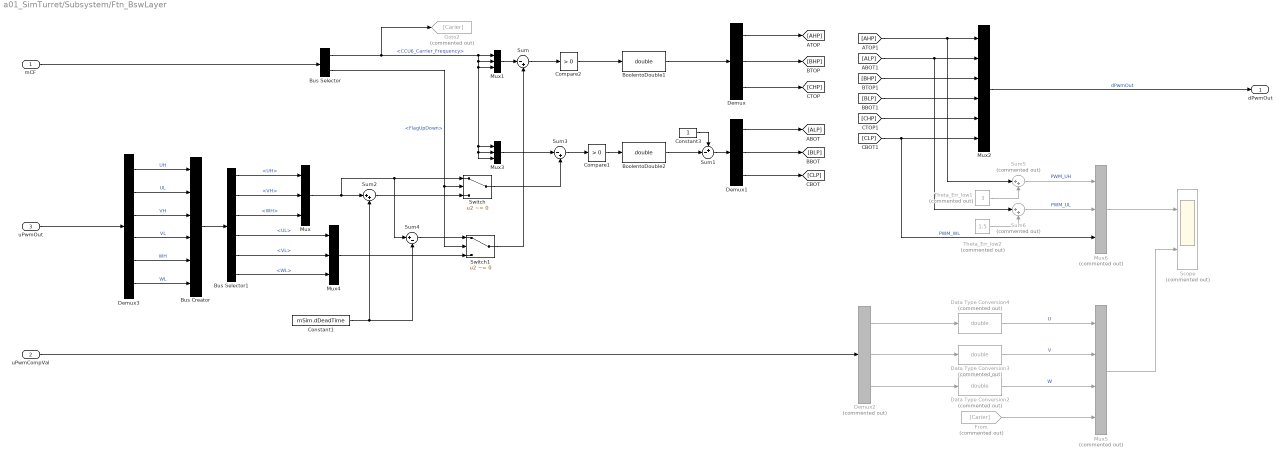
== system a01_SimTurret/Subsystem/Ftn_BswLayer ==
  mCF : Inport
  uPwmCompVal : Inport  Port=2
  uPwmOut : Inport  Port=3
  BoolentoDouble1 : DataTypeConversion  OutDataTypeStr=double  SaturateOnIntegerOverflow=off  RndMeth=Floor
  BoolentoDouble2 : DataTypeConversion  OutDataTypeStr=double  SaturateOnIntegerOverflow=off  RndMeth=Floor
  Bus Creator : BusCreator  Inputs=6
  Bus Selector : BusSelector  OutputSignals=CCU6_Carrier_Frequency,FlagUpDown
  Bus Selector1 : BusSelector  OutputSignals=UH,VH,WH,UL,VL,WL
  Compare1 : simulink/Logic and Bit Operations/Compare To Constant  relop=>  const=0  OutDataTypeStr=boolean
  Compare2 : simulink/Logic and Bit Operations/Compare To Constant  relop=>  const=0  OutDataTypeStr=boolean
  Constant1 : Constant  Value=mSim.dDeadTime
  Constant3 : Constant
  Data Type Conversion2 : DataTypeConversion  Commented=on  OutDataTypeStr=double  SaturateOnIntegerOverflow=off  RndMeth=Floor
  Data Type Conversion3 : DataTypeConversion  Commented=on  OutDataTypeStr=double  SaturateOnIntegerOverflow=off  RndMeth=Floor
  Data Type Conversion4 : DataTypeConversion  Commented=on  OutDataTypeStr=double  SaturateOnIntegerOverflow=off  RndMeth=Floor
  Demux : Demux  Outputs=3
  Demux1 : Demux  Outputs=3
  Demux2 : Demux  Commented=on  Outputs=3
  Demux3 : Demux  Outputs=6
  From : From  Commented=on  GotoTag=Carier
  Goto2 : Goto  Commented=on  GotoTag=Carier
  Mux{,1,3..4} (4 alike) : Mux  Inputs=3
  Mux2 : Mux  Inputs=6
  Mux5 : Mux  Commented=on
  Mux6 : Mux  Commented=on  Inputs=3
  Scope : Scope  Commented=on  NumInputPorts=2
  Sum : Sum  Inputs=|-+
  Sum1 : Sum  Inputs=+-|
  Sum2 : Sum  Inputs=|++
  Sum3 : Sum  Inputs=|-+
  Sum4 : Sum  Inputs=|+-
  Sum5 : Sum  Commented=on  Inputs=|++
  Sum6 : Sum  Commented=on  Inputs=|++
  Switch : Switch  Criteria=u2 ~= 0  SaturateOnIntegerOverflow=off  InputSameDT=off
  Switch1 : Switch  Criteria=u2 ~= 0  SaturateOnIntegerOverflow=off  InputSameDT=off
  Theta_Err_low1 : Constant  Commented=on  Value=3  OutDataTypeStr=double
  Theta_Err_low2 : Constant  Commented=on  Value=1.5  OutDataTypeStr=double
  dPwmOut : Outport
  wires:
  Mux3/1 -> Sum3/1
  uPwmCompVal/1 -> Demux2/1
  BoolentoDouble1/1 -> Demux/1
  Bus Creator/1 -> Bus Selector1/1
  Sum6/1 -> Mux6/2  "PWM_UL"
  Demux3/1 -> Bus Creator/1  "UH"
  Demux3/3 -> Bus Creator/3  "VH"
  [BHP] -> Mux2/3
  Sum/1 -> Compare2/1
  Demux3/4 -> Bus Creator/4  "VL"
  uPwmOut/1 -> Demux3/1
  Demux2/3 -> Data Type Conversion2/1
  Switch/1 -> Sum3/2
  Data Type Conversion4/1 -> Mux5/1  "U"
  Demux3/5 -> Bus Creator/5  "WH"
  Demux2/1 -> Data Type Conversion4/1
  Bus Selector/2 -> Switch1/2, Switch/2  "<FlagUpDown>"
  Demux/1 -> [AHP]
  From/1 -> Mux5/4
  Bus Selector1/4 -> Mux4/1  "<UL>"
  Data Type Conversion3/1 -> Mux5/2  "V"
  Demux3/6 -> Bus Creator/6  "WL"
  Demux1/1 -> [ALP]
  Bus Selector1/3 -> Mux/3  "<WH>"
  Demux/2 -> [BHP]
  [ALP] -> Sum6/1, Mux2/2
  Sum4/1 -> Switch1/1
  Constant1/1 -> Sum2/2, Sum4/2
  Switch1/1 -> Sum/2
  [BLP] -> Mux2/4
  Mux/1 -> Sum2/1, Sum4/1, Switch/1
  [CLP] -> Mux2/6, Mux6/3  "PWM_WL"
  Demux/3 -> [CHP]
  Bus Selector1/2 -> Mux/2  "<VH>"
  BoolentoDouble2/1 -> Sum1/2
  Demux1/2 -> [BLP]
  Mux2/1 -> dPwmOut/1  "dPwmOut"
  Mux1/1 -> Sum/1
  Sum3/1 -> Compare1/1
  Compare2/1 -> BoolentoDouble1/1
  mCF/1 -> Bus Selector/1
  Demux1/3 -> [CLP]
  Bus Selector1/5 -> Mux4/2  "<VL>"
  Bus Selector/1 -> Goto2/1, Mux1/1, Mux3/1, Mux3/3, Mux3/2, Mux1/3, Mux1/2  "<CCU6_Carrier_Frequency>"
  Theta_Err_low2/1 -> Sum6/2
  [AHP] -> Sum5/1, Mux2/1
  Theta_Err_low1/1 -> Sum5/2
  Demux2/2 -> Data Type Conversion3/1
  [CHP] -> Mux2/5
  Sum5/1 -> Mux6/1  "PWM_UH"
  Demux3/2 -> Bus Creator/2  "UL"
  Mux6/1 -> Scope/1
  Compare1/1 -> BoolentoDouble2/1
  Sum2/1 -> Switch/3
  Mux4/1 -> Switch1/3
  Data Type Conversion2/1 -> Mux5/3  "W"
  Bus Selector1/6 -> Mux4/3  "<WL>"
  Sum1/1 -> Demux1/1
  Constant3/1 -> Sum1/1
  Bus Selector1/1 -> Mux/1  "<UH>"
  Mux5/1 -> Scope/2

== system a01_SimTurret/Subsystem/Ftn_MtrCtrlPwmSet ==
  bC01MADC : Inport
  bE04GPWM : Inport  Port=2
  Trigger : TriggerPort  VariantControl=(inherit)  PortDimensions=1
  Bus Creator : BusCreator  Inputs=2
  Constant1 : Constant  Value=mSim.dPrdHalf  OutDataTypeStr=uint16
  Constant5 : Constant  Value=mSim.dPrd  OutDataTypeStr=uint16
  Data Type Conversion2 : DataTypeConversion  OutDataTypeStr=uint16  SaturateOnIntegerOverflow=off  RndMeth=Floor
  If : If  IfExpression=u1 == 1
  Merge : Merge  Tag=PWMOUT
  PWM_DEFAULT : Subsystem
      settings: RTWSystemCode=Nonreusable function  RTWFcnNameOpts=Use subsystem name
  PWM_FOUT : Subsystem
      settings: RTWSystemCode=Nonreusable function  RTWFcnNameOpts=Use subsystem name
  uPWMAction : Constant  OutDataTypeStr=uint16
  uPwmCompVal : Outport
  uPwmOut : Outport  Port=2
  wires:
  Constant1/1 -> Bus Creator/2  "uPrdHalf"
  If/1 -> PWM_FOUT/Action
  Bus Creator/1 -> PWM_DEFAULT/1(bTBC), PWM_FOUT/3(bTBC)  "bTBC"
  Data Type Conversion2/1 -> If/1
  bE04GPWM/1 -> PWM_FOUT/1(bE04GPWM)
  PWM_FOUT/2(PWM_OUT) -> Merge/1
  uPWMAction/1 -> Data Type Conversion2/1
  Merge/1 -> uPwmOut/1  "uPwmOut"
  PWM_FOUT/1(uPwmCompVal) -> uPwmCompVal/1
  If/2 -> PWM_DEFAULT/Action
  PWM_DEFAULT/1(PWM_OUT) -> Merge/2
  bC01MADC/1 -> PWM_FOUT/2(bC01MADC)
  Constant5/1 -> Bus Creator/1  "uPrd"

== system a01_SimTurret/Subsystem/Interrupt_BSW ==
  note: Carrier_Frequency
  Bus Creator1 : BusCreator  Inputs=7
  Pulse Generator : DiscretePulseGenerator  PulseType=Time based  Period=mSim.dTime  PulseWidth=0.5  PhaseDelay=mSim.dTime*0.52
  Pulse Generator1 : DiscretePulseGenerator  PulseType=Time based  Period=mSim.dTime  PulseWidth=50
  Pulse Generator2 : DiscretePulseGenerator  PulseType=Time based  Period=mSim.dTime*10  PulseWidth=0.1  PhaseDelay=mSim.dTime*0.54
  Pulse Generator3 : DiscretePulseGenerator  PulseType=Time based  Period=mSim.dTime*100  PulseWidth=0.01  PhaseDelay=mSim.dTime*0.56
  Pulse Generator4 : DiscretePulseGenerator  PulseType=Time based  Period=mSim.dTime  PulseWidth=50
  RepeatingSequence1 : simulink/Sources/Repeating Sequence  rep_seq_t=[0 mSim.dTime]  rep_seq_y=[0 mSim.dPrdQuter]
  RepeatingSequence2 : simulink/Sources/Repeating Sequence  rep_seq_t=[0 mSim.dTime*0.5 mSim.dTime]  rep_seq_y=[0 mSim.dPrd 0]
  mCF : Outport  VectorParamsAs1DForOutWhenUnconnected=off
  wires:
  RepeatingSequence1/1 -> Bus Creator1/1  "GTM_Carrier_Frequency"
  RepeatingSequence2/1 -> Bus Creator1/2  "CCU6_Carrier_Frequency"
  Bus Creator1/1 -> mCF/1  "mCF"
  Pulse Generator/1 -> Bus Creator1/5  "Interrupt"
  Pulse Generator1/1 -> Bus Creator1/4  "SOC"
  Pulse Generator2/1 -> Bus Creator1/6  "Interrupt_T10"
  Pulse Generator3/1 -> Bus Creator1/7  "Interrupt_T100"
  Pulse Generator4/1 -> Bus Creator1/3  "FlagUpDown"
